simulink model "rlc_serie"  (R2024b)
settings: Solver=VariableStepAuto  StartTime=0.0  StopTime=end_time  RelTol=1e-3
values from neighbouring files (symbols this model uses):
  A = [0 1/Cap; -1/L -R/L]    [init_es2.m]
  B = [0;1/L]    [init_es2.m]
  C = [1 0]    [init_es2.m]
  D = [0]    [init_es2.m]
  L = 10e-3    (= 0.01)    [init_es2.m]
  om = 1*10^3    (= 1000)    [init_es2.m]
  R = 1e3    (= 1000)    [init_es2.m]
  U = 10    [init_es2.m]
  x0 = [x1_0 x2_0]    [init_es2.m]
  x1_0 = 0    [init_es2.m]
undefined symbols (not defined in the file or in its folder): den, num
settings Model: Creator=jacoposini  LastModifiedBy=jacoposini

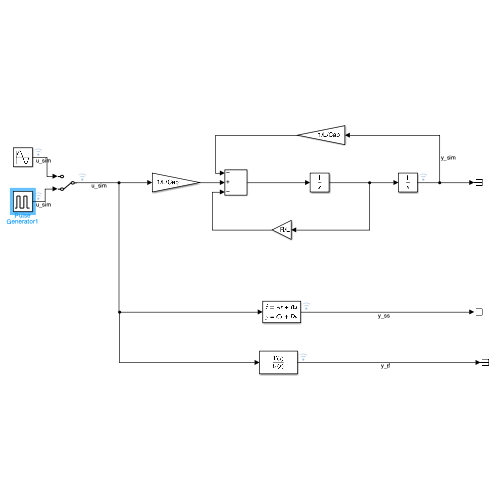
[thumbnail: Simulink's stored preview of the top-level diagram]
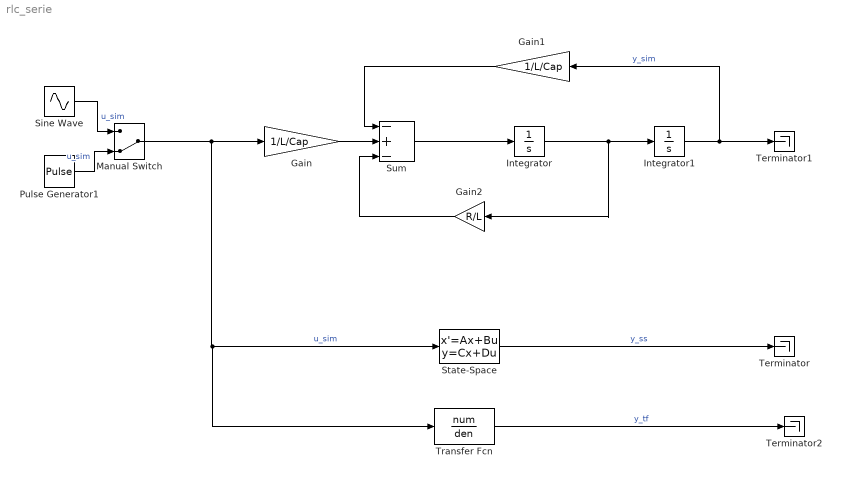
== system rlc_serie ==
  Gain : Gain  Gain=1/L/Cap
  Gain1 : Gain  Gain=1/L/Cap
  Gain2 : Gain  Gain=R/L
  Integrator : Integrator
  Integrator1 : Integrator  InitialCondition=x1_0
  Manual Switch : ManualSwitch  CurrentSetting=0
  Pulse Generator1 : DiscretePulseGenerator  PulseType=Time based  Amplitude=U  Period=2*pi/om  PulseWidth=50
  Sine Wave : Sin  Amplitude=U  Frequency=om  SampleTime=0
  State-Space : StateSpace  A=A  B=B  C=C  D=D  InitialCondition=x0
  Sum : Sum  Inputs=-+-
  Terminator : Terminator
  Terminator1 : Terminator
  Terminator2 : Terminator
  Transfer Fcn : TransferFcn  Numerator=num  Denominator=den
  wires:
  Gain/1 -> Sum/2
  Sum/1 -> Integrator/1
  Integrator/1 -> Gain2/1, Integrator1/1
  Integrator1/1 -> Terminator1/1, Gain1/1  "y_sim"
  Gain1/1 -> Sum/1
  Gain2/1 -> Sum/3
  State-Space/1 -> Terminator/1  "y_ss"
  Transfer Fcn/1 -> Terminator2/1  "y_tf"
  Manual Switch/1 -> Transfer Fcn/1, State-Space/1, Gain/1  "u_sim"
  Pulse Generator1/1 -> Manual Switch/2  "u_sim"
  Sine Wave/1 -> Manual Switch/1  "u_sim"
